simulink model "flightControlSystem"  (R2024b)
settings: Solver=ode3  StartTime=0  StopTime=TFinal  FixedStep=Ts  RelTol=1e-3  EnableMultiTasking=on
undefined symbols (not defined in the file): codertarget, Controller, DiscIntNeverNeededParam, Discrete, Estimator, g, init, K, Sensors, Time, Ts, var_acc_angle_N, var_bias_gyr_N, var_gyro_p_N, Vehicle
libraries: simulink x51, slpidlib x16, sharedtransform x5, ctrlSharedLib x3, eeGeneralControl x1, parrotlib x1
(part 5 of 5)

== matlab function flightControlSystem/Flight Control System/Controller1/SMC altitude controller/MATLAB Function ==
  data: z_d input; U1 output; z input; wd input; dz input; phi input; theta input; m input; w1 input; K input
function U1 = smc_altitude_control(z_d, z, wd, dz, phi, theta, m, w1, K)
    % SMC_ALTITUDE_CONTROL - Sliding Mode Control for altitude tracking
    % Inputs:
    %   z_d - Desired altitude
    %   Y7  - Measured altitude
    %   Y8  - Auxiliary state for disturbance observer
    %   phi - roll
    %   theta - pitch
    %   m   - Mass of the system
    %   g   - Gravitational acceleration
    %   lambda1 - Disturbance observer gain
    %   w1  - Positive constant for sliding surface
    % Output:
    %   U1  - Control input
       
    g = 9.81;
    % Tracking error
    e1 = z_d - z;
    
    % Sliding surface
    s1 = wd-dz + w1 * e1;
    
    
    % Control law (Equation 46 from the paper)
    U1 = (m / (cos(phi) * cos(theta))) * (z_d - g + w1 * e1 + K * tanh(s1));
end
